simulink model "UnitTest_relay_tripOutMng"  (Simulink 8.1)
settings: Solver=FixedStepDiscrete  StartTime=0.0  StopTime=16  FixedStep=Ts  RelTol=1e-3
PreLoadFcn:
  | Ts=100e-6;
InitFcn:
  | Ts=100e-6;
StartFcn:
  | Ts=100e-6;
libraries: simulink x3, relay_tripOutMng_lib x1
settings Model: Creator=re25624  LastModifiedBy=re25624
settings DataIOCC: SignalLoggingSaveFormat=Dataset
settings OptimizationCC: ExpressionDepthLimit=128
settings DebuggingCC: FcnCallInpInsideContextMsg=EnableAllAsError
settings GRTTargetCC: CombineOutputUpdateFcns=on  GRTInterface=off

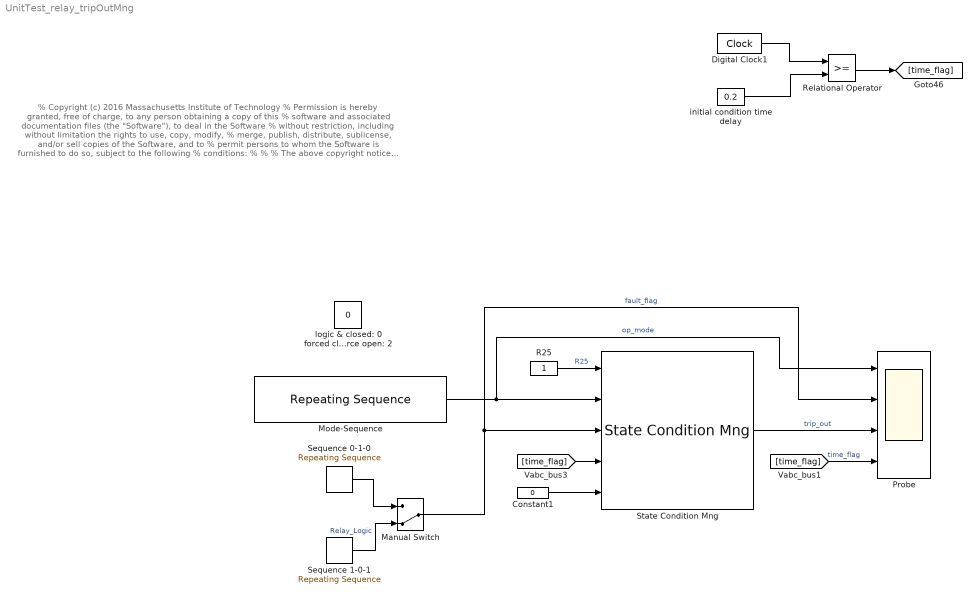
== system UnitTest_relay_tripOutMng ==
  note: % Copyright (c) 2016 Massachusetts Institute of Technology
      | % Permission is hereby granted, free of charge, to any person obtaining a copy of this
      | % software and associated documentation files (the "Software"), to deal in the Software
      | % without restriction, including without limitation the rights to use, copy, modify,
      | % merge, publish, distribute, sublicense, and/or sell copies of the Software, and to
      | % permit persons to whom the Software is furnished to do so, subject to the following
      | % conditions:
      | %
      | %
      | % The above copyright notice and this permission notice shall be included in
      | % all copies or substantial portions of the Software.
      | %
      | % THE SOFTWARE IS PROVIDED "AS IS", WITHOUT WARRANTY OF ANY KIND, EXPRESS OR IMPLIED,
      | % INCLUDING BUT NOT LIMITED TO THE WARRANTIES OF MERCHANTABILITY, FITNESS FOR A
      | % PARTICULAR PURPOSE AND NONINFRINGEMENT. IN NO EVENT SHALL THE AUTHORS OR COPYRIGHT
      | % HOLDERS BE LIABLE FOR ANY CLAIM, DAMAGES OR OTHER LIABILITY, WHETHER IN AN ACTION
      | % OF CONTRACT, TORT OR OTHERWISE, ARISING FROM, OUT OF OR IN CONNECTION WITH THE
      | % SOFTWARE OR THE USE OR OTHER DEALINGS IN THE SOFTWARE.
      | %
      | %
      | %%
  Constant1 : Constant  Value=0
  Digital Clock1 : DigitalClock  SampleTime=Ts
  Manual Switch : ManualSwitch  CurrentSetting=0
  Mode-Sequence : simulink/Sources/Repeating Sequence  rep_seq_t=|  rep_seq_y=|
      rep_seq_t=|
      | [0
      | 2
      | 2
      | 4
      | 4
      | 6
      | 6
      | 8
      | 8
      | 10
      | 10
      | 12
      | 12
      | 14
      | 14
      | 16]
      rep_seq_y=|
      | [0
      | 0
      | 1
      | 1
      | 0
      | 0
      | 2
      | 2
      | 1
      | 1
      | 0
      | 0
      | 2
      | 2
      | 0
      | 0]
  Probe : Scope  NumInputPorts=4
      settings: ShowLegends=on  TimeRange=16  YMin=-1~-1~-5~0  YMax=3~1.5~5~1
  R25 : Constant
  Relational Operator : RelationalOperator  OutDataTypeStr=boolean
  Sequence 0-1-0 : simulink/Sources/Repeating Sequence  rep_seq_t=[0 2.5 2.5 4.5 4.5 10]  rep_seq_y=[0 0 1 1 0 0]
  Sequence 1-0-1 : simulink/Sources/Repeating Sequence  rep_seq_t=[0 2.5 2.5 4.5 4.5 10]  rep_seq_y=[1 1 0 0 1 1]
  State Condition Mng : relay_tripOutMng_lib/State Condition Mng
  initial condition time delay : Constant  Value=0.2
  logic & closed: 0 forced closed: 1 force open: 2 : Constant  Value=0
  wires:
  Sequence 1-0-1/1 -> Manual Switch/2  "Relay_Logic"
  Sequence 0-1-0/1 -> Manual Switch/1
  Constant1/1 -> State Condition Mng/5
  Mode-Sequence/1 -> Probe/1, State Condition Mng/2  "op_mode"
  R25/1 -> State Condition Mng/1  "R25"
  Digital Clock1/1 -> Relational Operator/1
  initial condition time delay/1 -> Relational Operator/2
  Relational Operator/1 -> [time_flag]
  Manual Switch/1 -> State Condition Mng/3, Probe/2  "fault_flag"
  [time_flag] -> State Condition Mng/4
  State Condition Mng/1 -> Probe/3  "trip_out"
  [time_flag] -> Probe/4  "time_flag"
